simulink model "algebraic_model"  (R2023a)
settings: Solver=VariableStepAuto  StartTime=0.0  StopTime=10.0  MaxStep=Ts*0.001  MinStep=Ts*0.0001  RelTol=1e-3
values from neighbouring files (symbols this model uses):
  Ts = 0.05    [MPC_design_1.m]    (also in algebraic_design.m = 0.005)
libraries: cstblocks x2
settings Model: Creator=s331500  LastModifiedBy=s331500

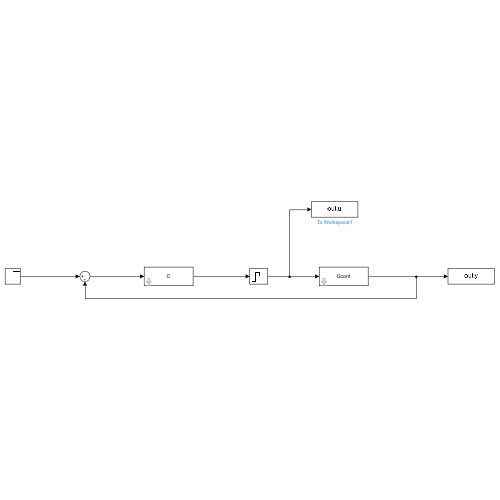
[thumbnail: Simulink's stored preview of the top-level diagram]
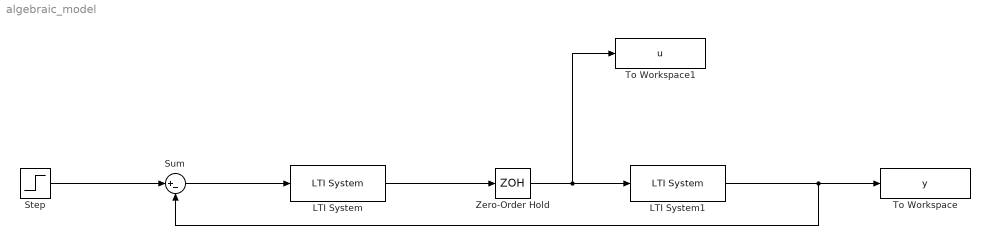
== system algebraic_model ==
  LTI System : cstblocks/LTI System  sys=C  IC=[]
  LTI System1 : cstblocks/LTI System  sys=Gcont  IC=[]
  Step : Step  Time=0  SampleTime=0
  Sum : Sum  Inputs=|+-
  To Workspace : ToWorkspace  VariableName=y  SaveFormat=Timeseries  SampleTime=Ts*0.001
  To Workspace1 : ToWorkspace  VariableName=u  SaveFormat=Timeseries  SampleTime=Ts*0.001
  Zero-Order Hold : ZeroOrderHold  SampleTime=Ts
  wires:
  Step/1 -> Sum/1
  Sum/1 -> LTI System/1
  LTI System/1 -> Zero-Order Hold/1
  Zero-Order Hold/1 -> To Workspace1/1, LTI System1/1
  LTI System1/1 -> Sum/2, To Workspace/1
